simulink model "px4demo_input_rc"  (R2017b)
settings: Solver=ode3  StartTime=0.0  StopTime=2  RelTol=1e-3  EnableMultiTasking=on
PostLoadFcn:
  | Ts = 1/250;
undefined symbols (not defined in the file or in its folder): RGBLED_COLOR_ENUM, RGBLED_MODE_ENUM
libraries: pixhawk_slib_sensors_actuators x2
Description:
  | PX4 PSP Example Model to show the RC Input Block working
  | 
  | Input RC Block Example
settings Model: Creator=skuznick  LastModifiedBy=skuznick
settings SolverCC: PositivePriorityOrder=on
settings DataIOCC: LimitDataPoints=on  SaveFormat=Array  SignalLoggingSaveFormat=ModelDataLogs
settings OptimizationCC: DefaultParameterBehavior=Inlined  LifeSpan=1  MaxStackSize=64
settings DebuggingCC: SolverPrmCheckMsg=warning  MultiTaskDSMMsg=warning  MultiTaskCondExecSysMsg=none  AllowSymbolicDim=off  SFUnexpectedBacktrackingDiag=warning  SFNoUnconditionalDefaultTransitionDiag=warning  SFExecutionAtInitializationDiag=none
settings HardwareCC: ProdBitPerPointer=32  ProdBitPerSizeT=32  ProdBitPerPtrDiffT=32  ProdLargestAtomicInteger=Long  ProdLargestAtomicFloat=Double  ProdWordSize=32  ProdHWDeviceType=ARM Compatible->ARM Cortex
settings ModelReferenceCC: PropagateSignalLabelsOutOfModel=off
settings SFSimCC: MATLABDynamicMemAlloc=off
settings RTWCC: SystemTargetFile=ert.tlc  HardwareBoard=Pixhawk PX4  TLCOptions="-aInlineSetEventsForThisBaseRateFcn=TLC_FALSE -aSuppressMultiTaskScheduler=TLC_FALSE    -aRateBasedStepFcn=0"  TemplateMakefile=ert_default_tmf  GenerateReport=on  Toolchain=Pixhawk Toolchain  BuildConfiguration=Faster Runs  IncludeHyperlinkInReport=on  LaunchReport=on  GenerateTraceReport=on  GenerateCodeMetricsReport=on
settings CodeAppCC: IgnoreCustomStorageClasses=off  StateflowObjectComments=on
settings ERTTargetCC: MultiwordLength=2048  ERTCustomFileTemplate=px4_codertarget_file_process.tlc  ConvertIfToSwitch=off  SuppressUnreachableDefaultCases=off
settings ConfigComp: CovMetricSettings=dw  CovHtmlReporting=on  CovSaveCumulativeToWorkspaceVar=on  CovSaveSingleToWorkspaceVar=on  CovExternalEMLEnable=off  CovSFcnEnable=off

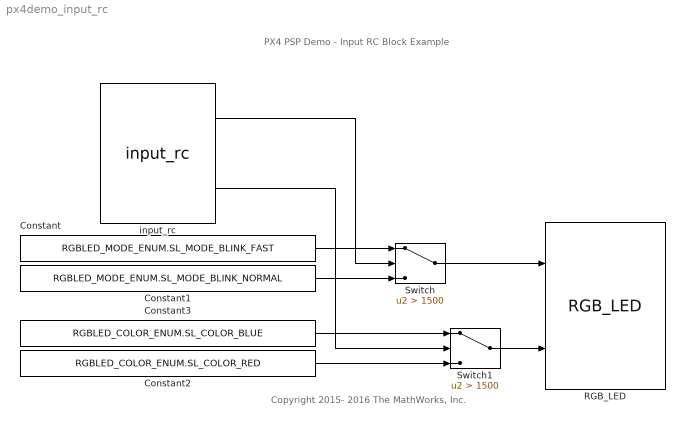
== system px4demo_input_rc ==
  note: PX4 PSP Demo - Input RC Block Example
  note: Copyright 2015- 2016 The MathWorks, Inc.
  Constant : Constant  Value=RGBLED_MODE_ENUM.SL_MODE_BLINK_FAST  OutDataTypeStr=Enum: RGBLED_MODE_ENUM
  Constant1 : Constant  Value=RGBLED_MODE_ENUM.SL_MODE_BLINK_NORMAL  OutDataTypeStr=Enum: RGBLED_MODE_ENUM
  Constant2 : Constant  Value=RGBLED_COLOR_ENUM.SL_COLOR_RED  OutDataTypeStr=Enum: RGBLED_COLOR_ENUM
  Constant3 : Constant  Value=RGBLED_COLOR_ENUM.SL_COLOR_BLUE  OutDataTypeStr=Enum: RGBLED_COLOR_ENUM
  RGB_LED : pixhawk_slib_sensors_actuators/RGB_LED
      settings: SourceProductName=Pixhawk Target Blocks
  Switch : Switch  Criteria=u2 > Threshold  Threshold=1500
  Switch1 : Switch  Criteria=u2 > Threshold  Threshold=1500
  input_rc : pixhawk_slib_sensors_actuators/input_rc  sampletime=Ts  channel1=off  channel2=off  channel3=on  channel4=on  channel5=off  channel6=off  channel7=off  channel8=off  channel9=off  channel10=off  channel11=off  channel12=off  channel13=off  channel14=off  channel15=off  channel16=off  channel17=off  channel18=off  ch_count=off  rssi=off  rc_failsafe=off  rc_lost=off  rc_inputsource=off
      settings: SourceProductName=Pixhawk Target Blocks
  wires:
  Switch/1 -> RGB_LED/1
  Switch1/1 -> RGB_LED/2
  Constant/1 -> Switch/1
  Constant1/1 -> Switch/3
  Constant3/1 -> Switch1/1
  Constant2/1 -> Switch1/3
  input_rc/1 -> Switch/2
  input_rc/2 -> Switch1/2
